simulink subsystem "SensoresVl53"  (R2023b)
settings: Solver=VariableStepAuto  StartTime=0.0  StopTime=10.0  RelTol=1e-3
settings Model: Creator=Hajar  LastModifiedBy=Hajar

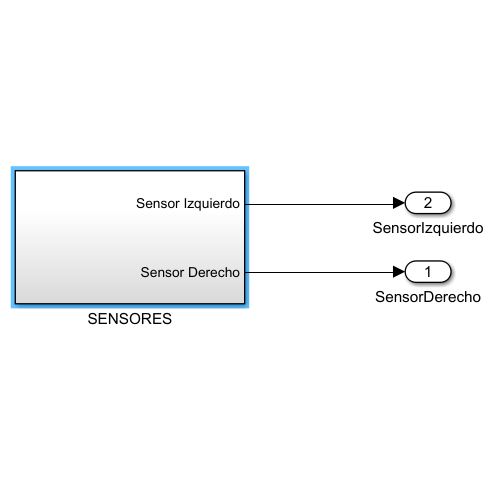
[thumbnail: Simulink's stored preview of the top-level diagram]
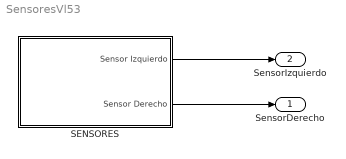
== system SensoresVl53 ==
  SENSORES : Subsystem
  SensorDerecho : Outport  VectorParamsAs1DForOutWhenUnconnected=off
  SensorIzquierdo : Outport  Port=2  VectorParamsAs1DForOutWhenUnconnected=off
  wires:
  SENSORES/2(Sensor Derecho) -> SensorDerecho/1
  SENSORES/1(Sensor Izquierdo) -> SensorIzquierdo/1

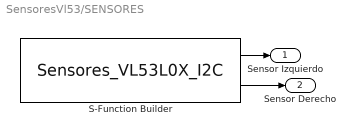
== system SensoresVl53/SENSORES ==
  S-Function Builder : S-Function  InitFcn=try, set_param(gcb,'FunctionName','Sensores_VL53L0X_I2C'), end  FunctionName=Sensores_VL53L0X_I2C  SFunctionModules=Sensores_VL53L0X_I2C_wrapper.c  SFunctionDeploymentMode=off  EnableBusSupport=off  mask(S-Function Builder){}
      mask help: Simulink:masks:SFunctionBuilder_MD
      mask init:
      | val = [[.9  0.75 0.75 1 1 .9 .9 1]',[1 1 0.75 0.75 .9 .9 1 .9]'];try , sys = get_param(gcb,'SfunBuilderFcnName');if isempty(sys), sys = get_param(gcb,'FunctionName'); end,catch, sys = get_param(gcb,'FunctionName'); end
      settings: CopyFcn=set_param(gcbh,'LinkStatus','none')  PreSaveFcn=try, set_param(gcb,'FunctionName','Sensores_VL53L0X_I2C'), end  OpenFcn=sfunctionwizard(gcbh)
      mask Display:
      | plot(val(:,1),val(:,2))
      | disp(sys)
      | port_label('output',1,'Sensor1')
      | port_label('output',2,'Sensor2')
  Sensor Izquierdo : Outport  VectorParamsAs1DForOutWhenUnconnected=off
  Sensor Derecho : Outport  Port=2  VectorParamsAs1DForOutWhenUnconnected=off
  wires:
  S-Function Builder/2 -> Sensor Derecho/1
  S-Function Builder/1 -> Sensor Izquierdo/1
